simulink model "UserDefinedModel"  (R2023b)
settings: Solver=ode45  StartTime=0.0  StopTime=20  MaxStep=0.001  RelTol=1e-3
libraries: spsSeriesRLCBranchLib x131, spsGroundLib x55, spsCurrentMeasurementLib x48, spsVoltageMeasurementLib x17, spsDiodeLib x4, spsControlledVoltageSourceLib x2, spspowerguiLib x1
(part 2 of 2)

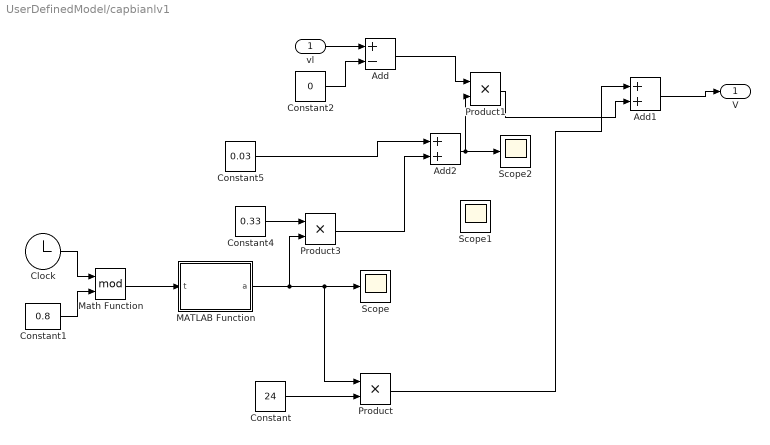
== system UserDefinedModel/capbianlv1 ==
  vl : Inport
  Add : Sum  Inputs=+-
  Add1 : Sum
  Add2 : Sum
  Clock : Clock
      settings: Decimation=1000
  Constant : Constant  Value=24
  Constant1 : Constant  Value=0.8
  Constant2 : Constant  Value=0
  Constant4 : Constant  Value=0.33
  Constant5 : Constant  Value=0.03
  MATLAB Function : MATLAB Function  TreatAsAtomicUnit=on
  Math Function : Math  Operator=mod  SignedPower=on
  Product : Product
  Product1 : Product
  Product3 : Product
  Scope : Scope
  Scope1 : Scope
  Scope2 : Scope
  V : Outport  VectorParamsAs1DForOutWhenUnconnected=off
  wires:
  Constant1/1 -> Math Function/2
  Math Function/1 -> MATLAB Function/1(t)
  Clock/1 -> Math Function/1
  MATLAB Function/1(a) -> Product/1, Scope/1, Product3/2
  Constant/1 -> Product/2
  Constant2/1 -> Add/2
  Add1/1 -> V/1
  Constant4/1 -> Product3/1
  Constant5/1 -> Add2/1
  Product/1 -> Add1/1
  vl/1 -> Add/1
  Add/1 -> Product1/1
  Add2/1 -> Scope2/1, Product1/2
  Product1/1 -> Add1/2
  Product3/1 -> Add2/2

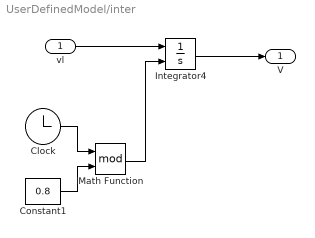
== system UserDefinedModel/inter ==
  vl : Inport
  Clock : Clock
  Constant1 : Constant  Value=0.8
  Integrator4 : Integrator  ExternalReset=falling  InitialCondition=150  UpperSaturationLimit=130  LowerSaturationLimit=60
  Math Function : Math  Operator=mod  SignedPower=on
  V : Outport  VectorParamsAs1DForOutWhenUnconnected=off
  wires:
  vl/1 -> Integrator4/1
  Clock/1 -> Math Function/1
  Constant1/1 -> Math Function/2
  Math Function/1 -> Integrator4/2
  Integrator4/1 -> V/1

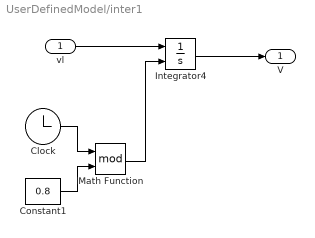
== system UserDefinedModel/inter1 ==
  vl : Inport
  Clock : Clock
  Constant1 : Constant  Value=0.8
  Integrator4 : Integrator  ExternalReset=falling  InitialCondition=150  UpperSaturationLimit=130  LowerSaturationLimit=60
  Math Function : Math  Operator=mod  SignedPower=on
  V : Outport  VectorParamsAs1DForOutWhenUnconnected=off
  wires:
  vl/1 -> Integrator4/1
  Clock/1 -> Math Function/1
  Constant1/1 -> Math Function/2
  Math Function/1 -> Integrator4/2
  Integrator4/1 -> V/1

== matlab function UserDefinedModel/capbianlv/MATLAB Function ==
  data: t input; a output
function a = fcn(t)
a=(1-cos(2*pi*t/0.4))/2.*(t<0.4);

== matlab function UserDefinedModel/capbianlv1/MATLAB Function ==
  data: t input; a output
function a = fcn(t)
a=(1-cos(2*pi*t/0.4))/2.*(t<=0.4);
